simulink model "CLLC_simu"  (R2025b)
settings: Solver=ode23tb  StartTime=0.0  StopTime=simlength  MaxStep=tc  RelTol=1e-3
values from neighbouring files (symbols this model uses):
  alpha1 = 0    [init.m]    (also in state_space_equations.m = linspace(pi/2,pi,3))
  alpha2 = 0    [init.m]    (also in state_space_equations.m = linspace(pi/2,pi,3))
  fr = 1/(2*pi*sqrt(Lr1*Cr1))    [init.m]
  phase_shift = pi/6    (= 0.523598775598)    [init.m]
  R1 = 0.026    [Optimal_Design_CLLLC.m]    (also in init.m = 0.1; state_space_equations.m = 0.1)
  R2 = 0.026    [Optimal_Design_CLLLC.m]    (also in init.m = 0.1; state_space_equations.m = 0.1)
  Td = 0.015 * Ts    (= 1.66666666667e-07)    [init.m]
libraries: fl_lib x60, nesl_utility x35, ee_lib x2, eeGeneralControl x1, single_phase_transformer x1
(part 1 of 2)
settings Model: SimulationMode=accelerator  Creator=i0013805  LastModifiedBy=torai

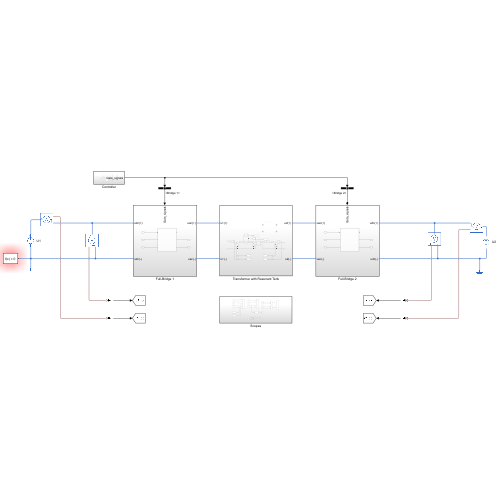
[thumbnail: Simulink's stored preview of the top-level diagram]
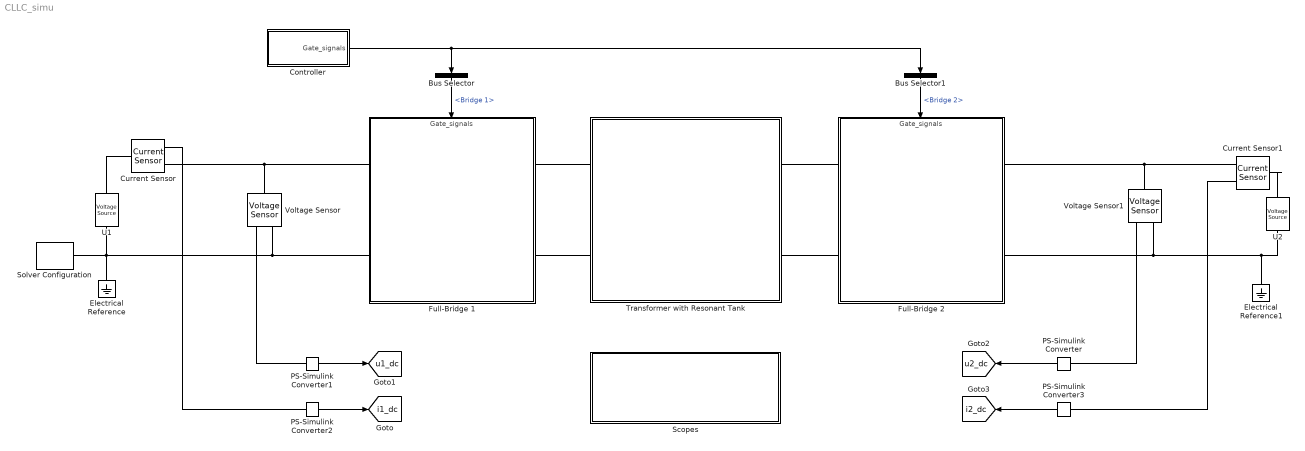
== system CLLC_simu ==
  Bus Selector : BusSelector  OutputSignals=Bridge 1
  Bus Selector1 : BusSelector  OutputSignals=Bridge 2
  Controller : Subsystem
  Current Sensor : fl_lib/Electrical/Electrical Sensors/Current Sensor
  Current Sensor1 : fl_lib/Electrical/Electrical Sensors/Current Sensor
  Electrical Reference : fl_lib/Electrical/Electrical Elements/Electrical Reference
  Electrical Reference1 : fl_lib/Electrical/Electrical Elements/Electrical Reference
  Full-Bridge 1 : Subsystem
      settings: PortSchema="{\"entries\":[{\"content\":{\"sides\":[{\"content\":{\"connectorIds\":[\"LConn1\",\"LConn2\"]},\"type\":\"ConnectorPlacement.EquallySpacedRectSide\",\"uuid\":\"3353105e-e30e-4d15-8630-1aa6d339e0ff\"},{\"content\":{\"connectorIds\":[\"RConn1\",\"RConn2\"],\"side\":\"RIGHT\"},\"type\":\"ConnectorPlacement.EquallySpacedRectSide\",\"uuid\":\"296f84bb-4176-46a6-993d-d3f03b5e0e3a\"},{\"content\":{\"connectorIds\":[\"In1\"],\"side\":\"TOP\"},\"type\":\"ConnectorPlacement.EquallySpacedRectSide\",\"uuid\":\"5e45aedc-9cf5-4fc9-baa6-17227fc5f4f5\"}]},\"type\":\"ConnectorPlacement.EquallySpacedConnector\",\"uuid\":\"c9e49bb0-57c4-4cc0-be60-b6700ac8c03a\"}],\"packageUris\":[\"http://schema.mathworks.com/mf0/Connector/R2020b\"],\"version\":\"1.0\"}"
  Full-Bridge 2 : Subsystem
      settings: PortSchema="{\"entries\":[{\"content\":{\"sides\":[{\"content\":{\"connectorIds\":[\"LConn1\",\"LConn2\"]},\"type\":\"ConnectorPlacement.EquallySpacedRectSide\",\"uuid\":\"3353105e-e30e-4d15-8630-1aa6d339e0ff\"},{\"content\":{\"connectorIds\":[\"RConn1\",\"RConn2\"],\"side\":\"RIGHT\"},\"type\":\"ConnectorPlacement.EquallySpacedRectSide\",\"uuid\":\"296f84bb-4176-46a6-993d-d3f03b5e0e3a\"},{\"content\":{\"connectorIds\":[\"In1\"],\"side\":\"TOP\"},\"type\":\"ConnectorPlacement.EquallySpacedRectSide\",\"uuid\":\"5e45aedc-9cf5-4fc9-baa6-17227fc5f4f5\"}]},\"type\":\"ConnectorPlacement.EquallySpacedConnector\",\"uuid\":\"c9e49bb0-57c4-4cc0-be60-b6700ac8c03a\"}],\"packageUris\":[\"http://schema.mathworks.com/mf0/Connector/R2020b\"],\"version\":\"1.0\"}"
  PS-Simulink Converter{,1..3} (4 alike) : nesl_utility/PS-Simulink Converter  PhysicalDomain=network_engine_domain  SubClassName=ps_output  LeftPortType=input  RightPortType=output  PseudoPeriodic=off  Frequencies=[]  VectorFormat=inherit  Unit=inherit  AffineConversion=off
  Scopes : Subsystem
  Solver Configuration : nesl_utility/Solver Configuration  PhysicalDomain=network_engine_domain  SubClassName=solver  LeftPortType=input  RightPortType=generic  Tones=[]  Harmonics=[]  SimulateNoise=off  Profile=off  UseLocalSampling=off  EnableSwitchedLinearOptims=on  FrequencyDomain=off  UseCCode=off  RelTol=0.001  AbsTol=0.001  MinStep=1e-09  ToWorkspace=off  RevertToSquareIcSolve=off  NumHomotopyIterations=100  PhasorMode=off  PhasorModeNumHarmonics=1  ConsistencySolver=NEWTON_XTOL_AFTER_FTOL  IndexReductionMethod=DerivativeReplacement  DoDC=off  ResidualTolerance=1e-09  ConsistencyTolSource=GLOBAL  ConsistencyAbsTol=0.001  ConsistencyRelTol=0.001  ConsistencyTolFactor=0.001  UseLocalSolver=on  LocalSolverChoice=NE_BACKWARD_EULER_ADVANCER  ResolveIndetEquations=on  FunctionEvalNumThread=1  LocalSolverSampleTime=tc  DoFixedCost=on  MaxNonlinIter=5  MaxModeIter=2  ComputeImpulses=off  ImpulseIterations=2  LinearAlgebra=auto  LinearAlgebraNumThread=0  EquationFormulation=NE_TIME_EF  DelaysMemoryBudget=1024  AutomaticFiltering=on  FilteringTimeConstant=0.001  PartitionStorageMethod=AS_NEEDED  PartitionMemoryBudget=1024  PartitionMethod=ROBUST  MultibodyUseLocalSolver=off  MultibodyLocalSolverChoice=ODE1  MultibodyLocalSolverSampleTime=0.001
  Transformer with Resonant Tank : Subsystem
  U1 : ee_lib/Sources/Voltage Source  dc_voltage=800 V  ac_voltage=0 V  ac_shift=0 rad  ac_frequency=60 Hz  noise_mode=ee.enum.sources.noise.Disabled  PSD=0 V^2/Hz  sample_time=1e-3 s  repeatability=ee.enum.sources.repeatability.NotRepeatable  user_seed=0  auto_seed=3499211588  i_specify=off  i_priority=None  i=0 A  i_nominal_specify=off  i_nominal_value=1  i_nominal_unit=A  v_specify=off  v_priority=None  v=0 V  v_nominal_specify=off  v_nominal_value=1  v_nominal_unit=V
  U2 : ee_lib/Sources/Voltage Source  dc_voltage=800 V  ac_voltage=0 V  ac_shift=0 rad  ac_frequency=60 Hz  noise_mode=ee.enum.sources.noise.Disabled  PSD=0 V^2/Hz  sample_time=1e-3 s  repeatability=ee.enum.sources.repeatability.NotRepeatable  user_seed=0  auto_seed=3890346746  i_specify=off  i_priority=None  i=0 A  i_nominal_specify=off  i_nominal_value=1  i_nominal_unit=A  v_specify=off  v_priority=None  v=0 V  v_nominal_specify=off  v_nominal_value=1  v_nominal_unit=V
  Voltage Sensor : fl_lib/Electrical/Electrical Sensors/Voltage Sensor
  Voltage Sensor1 : fl_lib/Electrical/Electrical Sensors/Voltage Sensor
  tag scope: i1_dc=global, i2_dc=global, u1_dc=global, u2_dc=global
  wires:
  Bus Selector/1 -> Full-Bridge 1/1(Gate_signals)  "<Bridge 1>"
  Controller/1(Gate_signals) -> Bus Selector1/1, Bus Selector/1
  Bus Selector1/1 -> Full-Bridge 2/1(Gate_signals)  "<Bridge 2>"
  PS-Simulink Converter2/1 -> [i1_dc]
  PS-Simulink Converter1/1 -> [u1_dc]
  PS-Simulink Converter/1 -> [u2_dc]
  PS-Simulink Converter3/1 -> [i2_dc]
  connections:
  U2/RConn1 -- Electrical Reference1/LConn1 -- Full-Bridge 2/LConn2 -- Voltage Sensor1/RConn2
  Voltage Sensor/LConn1 -- Current Sensor/RConn2 -- Full-Bridge 1/LConn1
  Full-Bridge 1/RConn1 -- Transformer with Resonant Tank/LConn1
  Full-Bridge 1/RConn2 -- Transformer with Resonant Tank/LConn2
  U1/RConn1 -- Electrical Reference/LConn1 -- Full-Bridge 1/LConn2 -- Voltage Sensor/RConn2 -- Solver Configuration/RConn1
  Voltage Sensor/RConn1 -- PS-Simulink Converter1/LConn1
  Voltage Sensor1/RConn1 -- PS-Simulink Converter/LConn1
  Current Sensor/LConn1 -- U1/LConn1
  PS-Simulink Converter2/LConn1 -- Current Sensor/RConn1
  PS-Simulink Converter3/LConn1 -- Current Sensor1/RConn1
  Full-Bridge 2/RConn1 -- Transformer with Resonant Tank/RConn1
  Transformer with Resonant Tank/RConn2 -- Full-Bridge 2/RConn2
  Current Sensor1/LConn1 -- U2/LConn1
  Full-Bridge 2/LConn1 -- Current Sensor1/RConn2 -- Voltage Sensor1/LConn1

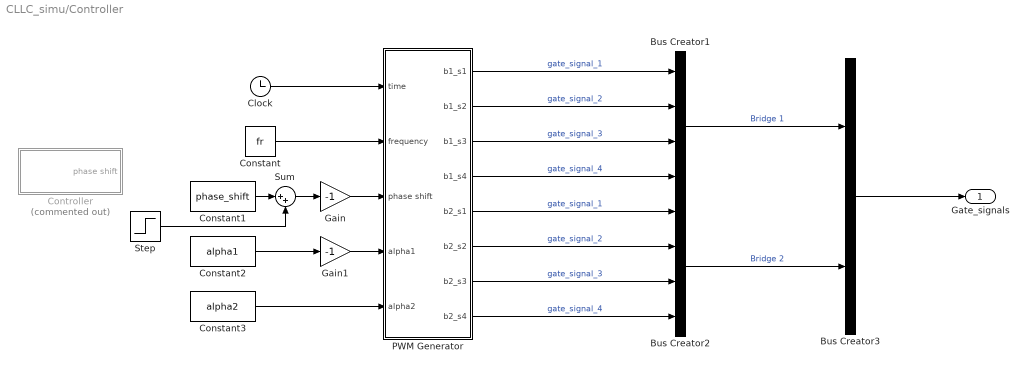
== system CLLC_simu/Controller ==
  Bus Creator1 : BusCreator  Inputs=4
  Bus Creator2 : BusCreator  Inputs=4
  Bus Creator3 : BusCreator  Inputs=2
  Clock : Clock
  Constant : Constant  Value=fr  VectorParams1D=off
  Constant1 : Constant  Value=phase_shift
  Constant2 : Constant  Value=alpha1
  Constant3 : Constant  Value=alpha2
  Controller : Subsystem  Commented=on
  Gain : Gain  Gain=-1
  Gain1 : Gain  Gain=-1
  PWM Generator : Subsystem
  Step : Step  Time=0.3  After=2*pi*0.04  SampleTime=0
  Sum : Sum  Inputs=|++
  Gate_signals : Outport
  wires:
  Bus Creator3/1 -> Gate_signals/1
  Bus Creator1/1 -> Bus Creator3/1  "Bridge 1"
  Bus Creator2/1 -> Bus Creator3/2  "Bridge 2"
  PWM Generator/1(b1_s1) -> Bus Creator1/1  "gate_signal_1"
  PWM Generator/4(b1_s4) -> Bus Creator1/4  "gate_signal_4"
  PWM Generator/2(b1_s2) -> Bus Creator1/2  "gate_signal_2"
  PWM Generator/3(b1_s3) -> Bus Creator1/3  "gate_signal_3"
  PWM Generator/5(b2_s1) -> Bus Creator2/1  "gate_signal_1"
  PWM Generator/6(b2_s2) -> Bus Creator2/2  "gate_signal_2"
  PWM Generator/7(b2_s3) -> Bus Creator2/3  "gate_signal_3"
  PWM Generator/8(b2_s4) -> Bus Creator2/4  "gate_signal_4"
  Clock/1 -> PWM Generator/1(time)
  Constant/1 -> PWM Generator/2(frequency)
  Constant2/1 -> Gain1/1
  Constant3/1 -> PWM Generator/5(alpha2)
  Gain/1 -> PWM Generator/3(phase shift)
  Gain1/1 -> PWM Generator/4(alpha1)
  Constant1/1 -> Sum/1
  Sum/1 -> Gain/1
  Step/1 -> Sum/2

== system CLLC_simu/Full-Bridge 1 ==
  Gate_signals : Inport
  Full-Bridge Ideal Switches : Subsystem
  udc(+) : PMIOPort  Side=Left
  udc(-) : PMIOPort  Port=2  Side=Left
  uac(+) : PMIOPort  Port=3  Side=Right
  uac(-) : PMIOPort  Port=4  Side=Right
  wires:
  Gate_signals/1 -> Full-Bridge Ideal Switches/1(Gate_signals)
  connections:
  udc(-)/RConn1 -- Full-Bridge Ideal Switches/LConn2
  Full-Bridge Ideal Switches/RConn1 -- uac(+)/RConn1
  Full-Bridge Ideal Switches/RConn2 -- uac(-)/RConn1
  udc(+)/RConn1 -- Full-Bridge Ideal Switches/LConn1

== system CLLC_simu/Full-Bridge 2 ==
  Gate_signals : Inport
  Full-Bridge Ideal Switches : Subsystem
  udc(+) : PMIOPort  Side=Left
  udc(-) : PMIOPort  Port=2  Side=Left
  uac(+) : PMIOPort  Port=3  Side=Right
  uac(-) : PMIOPort  Port=4  Side=Right
  wires:
  Gate_signals/1 -> Full-Bridge Ideal Switches/1(Gate_signals)
  connections:
  udc(-)/RConn1 -- Full-Bridge Ideal Switches/LConn2
  Full-Bridge Ideal Switches/RConn1 -- uac(+)/RConn1
  Full-Bridge Ideal Switches/RConn2 -- uac(-)/RConn1
  udc(+)/RConn1 -- Full-Bridge Ideal Switches/LConn1

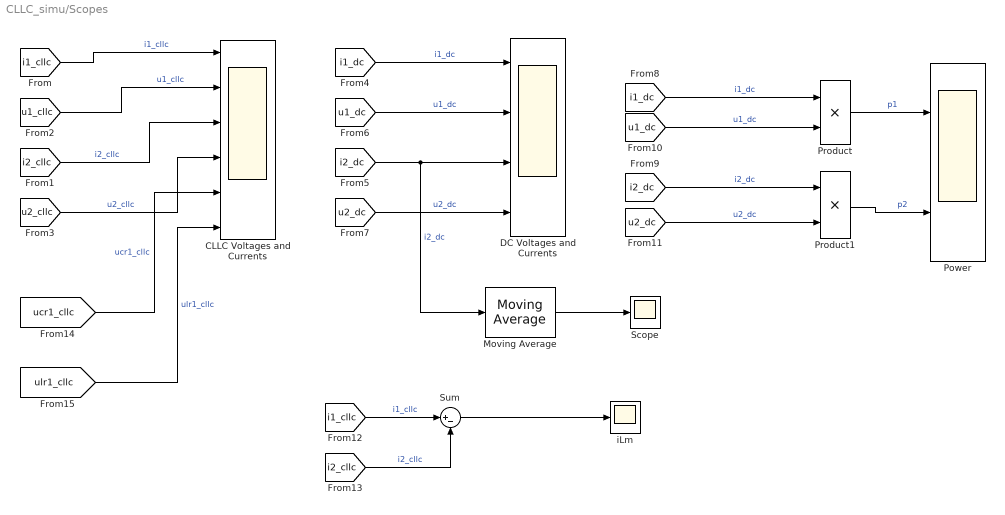
== system CLLC_simu/Scopes ==
  CLLC Voltages and Currents : Scope  NumInputPorts=6
      settings: ActiveDisplayYMinimum=-1023.9248688451665  ActiveDisplayYMaximum=1024.1887494959194
  DC Voltages and Currents : Scope  NumInputPorts=4
      settings: ActiveDisplayString=4  ActiveDisplayYMinimum=9  ActiveDisplayYMaximum=29
  Moving Average : eeGeneralControl/Moving Average  VariantControl=Variant1  LabelModeActiveChoice=Discrete  f=100e3  x0=0  BufferSize=8192  Ts=-1
      settings: LibrarySourceBlock=ee_sl_lib/General Control/Moving Average
  Power : Scope  NumInputPorts=2
      settings: ActiveDisplayYMinimum=-2.5651019732390419E+6  ActiveDisplayYMaximum=1.2445984514162283E+7  DataLoggingVariableName=ScopeData2
  Product : Product
  Product1 : Product
  Scope : Scope
      settings: ActiveDisplayYMinimum=-3.0858146971641012  ActiveDisplayYMaximum=-1.209999064201392  DataLoggingVariableName=ScopeData4
  Sum : Sum  Inputs=|+-
  iLm : Scope
      settings: ActiveDisplayYMinimum=-41.350666404493246  ActiveDisplayYMaximum=41.348326835244379  DataLoggingVariableName=ScopeData3
  wires:
  [i1_cllc] -> CLLC Voltages and Currents/1  "i1_cllc"
  [u1_cllc] -> CLLC Voltages and Currents/2  "u1_cllc"
  [i2_cllc] -> CLLC Voltages and Currents/3  "i2_cllc"
  [u2_cllc] -> CLLC Voltages and Currents/4  "u2_cllc"
  [i1_dc] -> DC Voltages and Currents/1  "i1_dc"
  [u1_dc] -> DC Voltages and Currents/2  "u1_dc"
  [i2_dc] -> Moving Average/1, DC Voltages and Currents/3  "i2_dc"
  [u2_dc] -> DC Voltages and Currents/4  "u2_dc"
  [i1_dc] -> Product/1  "i1_dc"
  [i2_dc] -> Product1/1  "i2_dc"
  [u1_dc] -> Product/2  "u1_dc"
  Product/1 -> Power/1  "p1"
  Product1/1 -> Power/2  "p2"
  [u2_dc] -> Product1/2  "u2_dc"
  [i1_cllc] -> Sum/1  "i1_cllc"
  [i2_cllc] -> Sum/2  "i2_cllc"
  Sum/1 -> iLm/1
  Moving Average/1 -> Scope/1
  [ucr1_cllc] -> CLLC Voltages and Currents/5  "ucr1_cllc"
  [ulr1_cllc] -> CLLC Voltages and Currents/6  "ulr1_cllc"

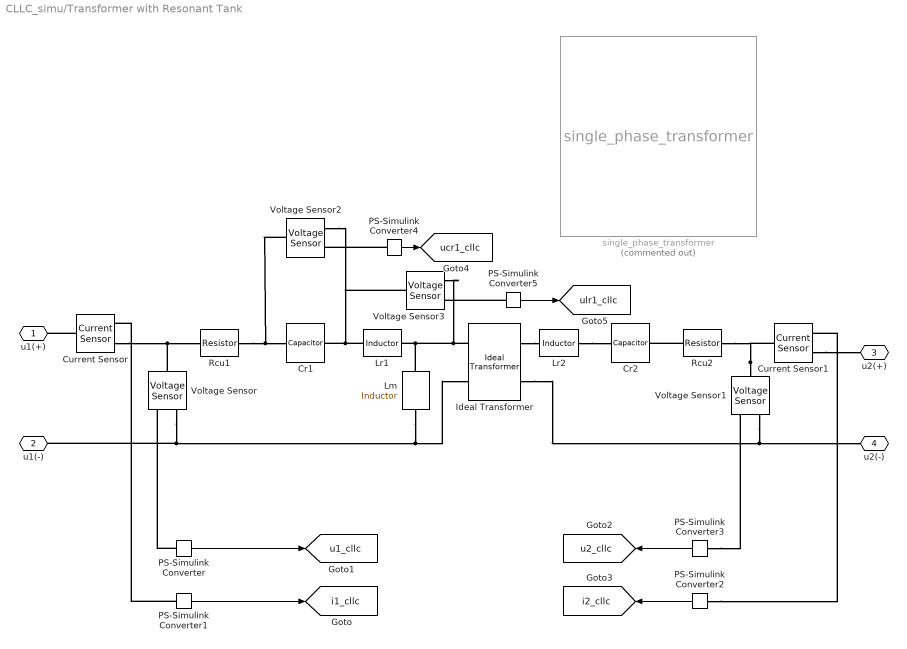
== system CLLC_simu/Transformer with Resonant Tank ==
  Cr1 : fl_lib/Electrical/Electrical Elements/Capacitor  c=Cr1 F  r=1e-6 Ohm  g=0 1/Ohm  i_specify=off  i_priority=None  i=0 A  i_nominal_specify=off  i_nominal_value=1  i_nominal_unit=A  v_specify=off  v_priority=None  v=0 V  v_nominal_specify=off  v_nominal_value=1  v_nominal_unit=V  vc_specify=off  vc_priority=High  vc=0 V  vc_nominal_specify=off  vc_nominal_value=1  vc_nominal_unit=V
  Cr2 : fl_lib/Electrical/Electrical Elements/Capacitor  c=Cr2 F  r=1e-6 Ohm  g=0 1/Ohm  i_specify=off  i_priority=None  i=0 A  i_nominal_specify=off  i_nominal_value=1  i_nominal_unit=A  v_specify=off  v_priority=None  v=0 V  v_nominal_specify=off  v_nominal_value=1  v_nominal_unit=V  vc_specify=off  vc_priority=High  vc=0 V  vc_nominal_specify=off  vc_nominal_value=1  vc_nominal_unit=V
  Current Sensor : fl_lib/Electrical/Electrical Sensors/Current Sensor
  Current Sensor1 : fl_lib/Electrical/Electrical Sensors/Current Sensor
  Ideal Transformer : fl_lib/Electrical/Electrical Elements/Ideal Transformer  n=1  i1_specify=off  i1_priority=None  i1=0 A  i1_nominal_specify=off  i1_nominal_value=1  i1_nominal_unit=A  v1_specify=off  v1_priority=None  v1=0 V  v1_nominal_specify=off  v1_nominal_value=1  v1_nominal_unit=V  i2_specify=off  i2_priority=None  i2=0 A  i2_nominal_specify=off  i2_nominal_value=1  i2_nominal_unit=A  v2_specify=off  v2_priority=None  v2=0 V  v2_nominal_specify=off  v2_nominal_value=1  v2_nominal_unit=V
  Lm : fl_lib/Electrical/Electrical Elements/Inductor  l=Lm H  r=0 Ohm  g=1e-9 1/Ohm  i_specify=off  i_priority=None  i=0 A  i_nominal_specify=off  i_nominal_value=1  i_nominal_unit=A  v_specify=off  v_priority=None  v=0 V  v_nominal_specify=off  v_nominal_value=1  v_nominal_unit=V  i_L_specify=off  i_L_priority=High  i_L=0 A  i_L_nominal_specify=off  i_L_nominal_value=1  i_L_nominal_unit=A
  Lr1 : fl_lib/Electrical/Electrical Elements/Inductor  l=Lr1 H  r=0 Ohm  g=1e-9 1/Ohm  i_specify=off  i_priority=None  i=0 A  i_nominal_specify=off  i_nominal_value=1  i_nominal_unit=A  v_specify=off  v_priority=None  v=0 V  v_nominal_specify=off  v_nominal_value=1  v_nominal_unit=V  i_L_specify=off  i_L_priority=High  i_L=0 A  i_L_nominal_specify=off  i_L_nominal_value=1  i_L_nominal_unit=A
  Lr2 : fl_lib/Electrical/Electrical Elements/Inductor  l=Lr2 H  r=0 Ohm  g=1e-9 1/Ohm  i_specify=off  i_priority=None  i=0 A  i_nominal_specify=off  i_nominal_value=1  i_nominal_unit=A  v_specify=off  v_priority=None  v=0 V  v_nominal_specify=off  v_nominal_value=1  v_nominal_unit=V  i_L_specify=off  i_L_priority=High  i_L=0 A  i_L_nominal_specify=off  i_L_nominal_value=1  i_L_nominal_unit=A
  PS-Simulink Converter{,1..5} (6 alike) : nesl_utility/PS-Simulink Converter  PhysicalDomain=network_engine_domain  SubClassName=ps_output  LeftPortType=input  RightPortType=output  PseudoPeriodic=off  Frequencies=[]  VectorFormat=inherit  Unit=inherit  AffineConversion=off
  Rcu1 : fl_lib/Electrical/Electrical Elements/Resistor  R=R1 Ohm  i_specify=off  i_priority=None  i=0 A  i_nominal_specify=off  i_nominal_value=1  i_nominal_unit=A  v_specify=off  v_priority=None  v=0 V  v_nominal_specify=off  v_nominal_value=1  v_nominal_unit=V
  Rcu2 : fl_lib/Electrical/Electrical Elements/Resistor  R=R2 Ohm  i_specify=off  i_priority=None  i=0 A  i_nominal_specify=off  i_nominal_value=1  i_nominal_unit=A  v_specify=off  v_priority=None  v=0 V  v_nominal_specify=off  v_nominal_value=1  v_nominal_unit=V
  Voltage Sensor{,1..3} (4 alike) : fl_lib/Electrical/Electrical Sensors/Voltage Sensor
  single_phase_transformer : single_phase_transformer/single_phase_transformer  Commented=on  lm_trafo=L_m  m1=N1  m2=N2  rd1_trafo=R1  rd2_trafo=R2  ld1_trafo=Lr1  ld2_trafo=Lr2  rfe_trafo=Rfe  length_core=0.1  mu0=1.256637e-6  mur=mur
  u1(+) : PMIOPort  Side=Left
  u1(-) : PMIOPort  Port=2  Side=Left
  u2(+) : PMIOPort  Port=3  Side=Right
  u2(-) : PMIOPort  Port=4  Side=Right
  tag scope: i1_cllc=global, i2_cllc=global, u1_cllc=global, u2_cllc=global, ucr1_cllc=global, ulr1_cllc=global
  wires:
  PS-Simulink Converter1/1 -> [i1_cllc]
  PS-Simulink Converter/1 -> [u1_cllc]
  PS-Simulink Converter3/1 -> [u2_cllc]
  PS-Simulink Converter2/1 -> [i2_cllc]
  PS-Simulink Converter4/1 -> [ucr1_cllc]
  PS-Simulink Converter5/1 -> [ulr1_cllc]
  connections:
  Lr2/RConn1 -- Cr2/RConn1
  Lr1/LConn1 -- Voltage Sensor3/LConn1 -- Voltage Sensor2/RConn2 -- Cr1/RConn1
  Voltage Sensor1/RConn2 -- Ideal Transformer/RConn2 -- u2(-)/RConn1
  Voltage Sensor/LConn1 -- Current Sensor/RConn2 -- Rcu1/LConn1
  Voltage Sensor/RConn2 -- Lm/RConn1 -- Ideal Transformer/LConn2 -- u1(-)/RConn1
  Rcu2/RConn1 -- Cr2/LConn1
  PS-Simulink Converter/LConn1 -- Voltage Sensor/RConn1
  Current Sensor/LConn1 -- u1(+)/RConn1
  PS-Simulink Converter1/LConn1 -- Current Sensor/RConn1
  Current Sensor1/RConn2 -- u2(+)/RConn1
  PS-Simulink Converter3/LConn1 -- Voltage Sensor1/RConn1
  PS-Simulink Converter2/LConn1 -- Current Sensor1/RConn1
  Ideal Transformer/LConn1 -- Voltage Sensor3/RConn2 -- Lm/LConn1 -- Lr1/RConn1
  Ideal Transformer/RConn1 -- Lr2/LConn1
  PS-Simulink Converter4/LConn1 -- Voltage Sensor2/RConn1
  PS-Simulink Converter5/LConn1 -- Voltage Sensor3/RConn1
  Rcu1/RConn1 -- Voltage Sensor2/LConn1 -- Cr1/LConn1
  Voltage Sensor1/LConn1 -- Current Sensor1/LConn1 -- Rcu2/LConn1

== system CLLC_simu/Controller/Controller ==
  Constant : Constant
  Gain : Gain  Gain=1/(200e3/800)
  Gain1 : Gain  Gain=-1
  Quantizer : Quantizer  QuantizationInterval=0.00048828
  Subsystem : Subsystem
  Sum : Sum  Inputs=|+-
  Unit Delay2 : UnitDelay  SampleTime=-1  HasFrameUpgradeWarning=on
  Zero-Order Hold2 : ZeroOrderHold  SampleTime=-1
  phase shift : Outport
  wires:
  Constant/1 -> Sum/1
  [i2_dc] -> Gain/1
  Gain/1 -> Quantizer/1
  Quantizer/1 -> Zero-Order Hold2/1
  Zero-Order Hold2/1 -> Sum/2
  Gain1/1 -> Unit Delay2/1
  Sum/1 -> Subsystem/1(In1)
  Subsystem/1(Out1) -> Gain1/1
  Unit Delay2/1 -> phase shift/1

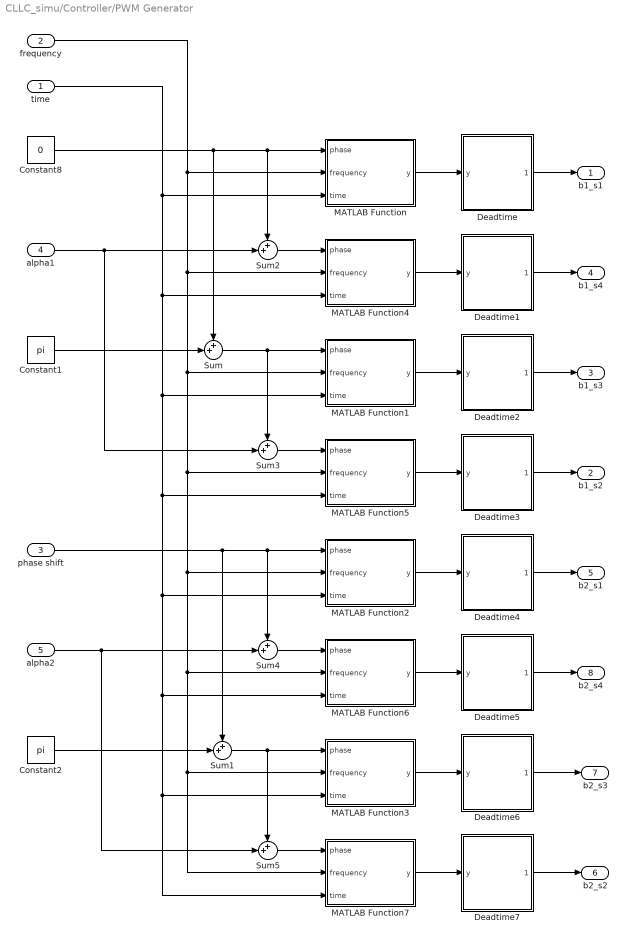
== system CLLC_simu/Controller/PWM Generator ==
  time : Inport
  frequency : Inport  Port=2
  phase shift : Inport  Port=3
  alpha1 : Inport  Port=4
  alpha2 : Inport  Port=5
  Constant1 : Constant  Value=pi
  Constant2 : Constant  Value=pi
  Constant8 : Constant  Value=0
  Deadtime : Subsystem
  Deadtime1 : Subsystem
  Deadtime2 : Subsystem
  Deadtime3 : Subsystem
  Deadtime4 : Subsystem
  Deadtime5 : Subsystem
  Deadtime6 : Subsystem
  Deadtime7 : Subsystem
  MATLAB Function : MATLAB Function  TreatAsAtomicUnit=on
  MATLAB Function1 : MATLAB Function  TreatAsAtomicUnit=on
  MATLAB Function2 : MATLAB Function  TreatAsAtomicUnit=on
  MATLAB Function3 : MATLAB Function  TreatAsAtomicUnit=on
  MATLAB Function4 : MATLAB Function  TreatAsAtomicUnit=on
  MATLAB Function5 : MATLAB Function  TreatAsAtomicUnit=on
  MATLAB Function6 : MATLAB Function  TreatAsAtomicUnit=on
  MATLAB Function7 : MATLAB Function  TreatAsAtomicUnit=on
  Sum{,1..5} (6 alike) : Sum  Inputs=++|
  b1_s1 : Outport
  b1_s2 : Outport  Port=2
  b1_s3 : Outport  Port=3
  b1_s4 : Outport  Port=4
  b2_s1 : Outport  Port=5
  b2_s2 : Outport  Port=6
  b2_s3 : Outport  Port=7
  b2_s4 : Outport  Port=8
  wires:
  Constant8/1 -> Sum/1, Sum2/1, MATLAB Function/1(phase)
  frequency/1 -> MATLAB Function5/2(frequency), MATLAB Function7/2(frequency), MATLAB Function3/2(frequency), MATLAB Function6/2(frequency), MATLAB Function2/2(frequency), MATLAB Function1/2(frequency), MATLAB Function4/2(frequency), MATLAB Function/2(frequency)
  time/1 -> MATLAB Function5/3(time), MATLAB Function3/3(time), MATLAB Function7/3(time), MATLAB Function6/3(time), MATLAB Function2/3(time), MATLAB Function1/3(time), MATLAB Function4/3(time), MATLAB Function/3(time)
  Sum/1 -> MATLAB Function1/1(phase), Sum3/1
  phase shift/1 -> Sum1/1, Sum4/1, MATLAB Function2/1(phase)
  Sum1/1 -> Sum5/1, MATLAB Function3/1(phase)
  MATLAB Function/1(y) -> Deadtime/1(y)
  Deadtime/1(1) -> b1_s1/1
  MATLAB Function1/1(y) -> Deadtime2/1(y)
  MATLAB Function2/1(y) -> Deadtime4/1(y)
  Deadtime5/1(1) -> b2_s4/1
  MATLAB Function3/1(y) -> Deadtime6/1(y)
  Deadtime6/1(1) -> b2_s3/1
  Deadtime7/1(1) -> b2_s2/1
  Constant1/1 -> Sum/2
  Constant2/1 -> Sum1/2
  Deadtime3/1(1) -> b1_s2/1
  alpha1/1 -> Sum3/2, Sum2/2
  Sum2/1 -> MATLAB Function4/1(phase)
  MATLAB Function4/1(y) -> Deadtime1/1(y)
  Deadtime1/1(1) -> b1_s4/1
  Sum3/1 -> MATLAB Function5/1(phase)
  MATLAB Function5/1(y) -> Deadtime3/1(y)
  Deadtime2/1(1) -> b1_s3/1
  Sum4/1 -> MATLAB Function6/1(phase)
  alpha2/1 -> Sum5/2, Sum4/2
  Deadtime4/1(1) -> b2_s1/1
  MATLAB Function6/1(y) -> Deadtime5/1(y)
  MATLAB Function7/1(y) -> Deadtime7/1(y)
  Sum5/1 -> MATLAB Function7/1(phase)

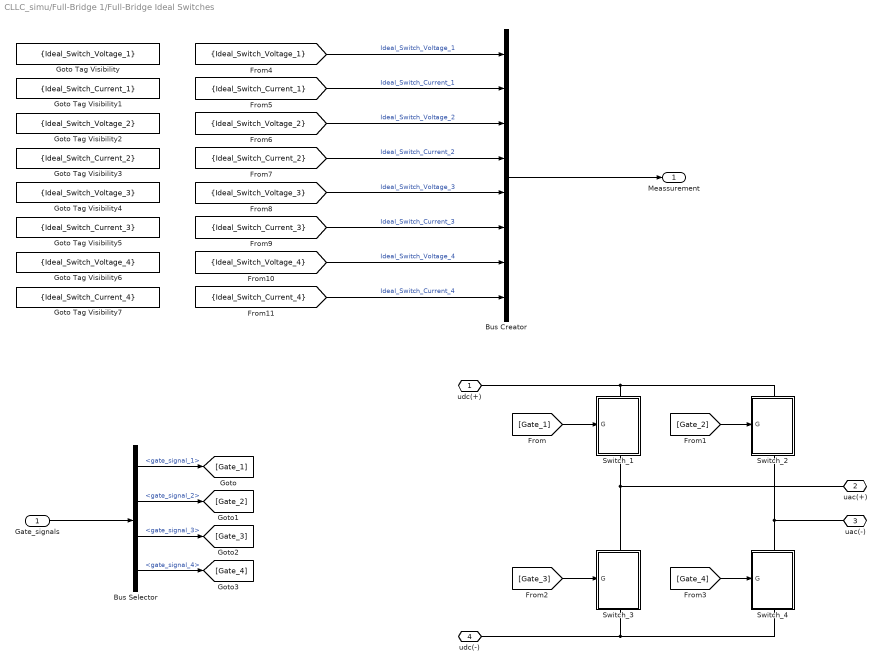
== system CLLC_simu/Full-Bridge 1/Full-Bridge Ideal Switches ==
  Gate_signals : Inport
  Bus Creator : BusCreator  Inputs=8
  Bus Selector : BusSelector  OutputSignals=gate_signal_1,gate_signal_2,gate_signal_3,gate_signal_4
  Goto Tag Visibility : GotoTagVisibility  GotoTag=Ideal_Switch_Voltage_1
  Goto Tag Visibility1 : GotoTagVisibility  GotoTag=Ideal_Switch_Current_1
  Goto Tag Visibility2 : GotoTagVisibility  GotoTag=Ideal_Switch_Voltage_2
  Goto Tag Visibility3 : GotoTagVisibility  GotoTag=Ideal_Switch_Current_2
  Goto Tag Visibility4 : GotoTagVisibility  GotoTag=Ideal_Switch_Voltage_3
  Goto Tag Visibility5 : GotoTagVisibility  GotoTag=Ideal_Switch_Current_3
  Goto Tag Visibility6 : GotoTagVisibility  GotoTag=Ideal_Switch_Voltage_4
  Goto Tag Visibility7 : GotoTagVisibility  GotoTag=Ideal_Switch_Current_4
  Switch_1 : Subsystem
      settings: PortSchema="{\"entries\":[{\"content\":{\"sides\":[{\"content\":{\"connectorIds\":[\"In1\"]},\"type\":\"ConnectorPlacement.EquallySpacedRectSide\",\"uuid\":\"812df248-72cf-4017-9d54-aef7207fce7f\"},{\"content\":{\"side\":\"RIGHT\"},\"type\":\"ConnectorPlacement.EquallySpacedRectSide\",\"uuid\":\"a66e31eb-6559-4312-afa0-26cb116d02bf\"},{\"content\":{\"connectorIds\":[\"LConn1\"],\"side\":\"TOP\"},\"type\":\"ConnectorPlacement.EquallySpacedRectSide\",\"uuid\":\"1df6feb4-8a8d-441a-a0dc-721a2bb21abb\"},{\"content\":{\"connectorIds\":[\"RConn1\"],\"side\":\"BOTTOM\"},\"type\":\"ConnectorPlacement.EquallySpacedRectSide\",\"uuid\":\"258c1e92-2fe7-4acf-9dd0-9c6d3fd42034\"}]},\"type\":\"ConnectorPlacement.EquallySpacedConnector\",\"uuid\":\"c9b0d122-031a-4b9b-b90c-c03d042c7b1a\"}],\"packageUris\":[\"http://schema.mathworks.com/mf0/Connector/R2020b\"],\"version\":\"1.0\"}"
  Switch_2 : Subsystem
      settings: PortSchema="{\"entries\":[{\"content\":{\"sides\":[{\"content\":{\"connectorIds\":[\"In1\"]},\"type\":\"ConnectorPlacement.EquallySpacedRectSide\",\"uuid\":\"812df248-72cf-4017-9d54-aef7207fce7f\"},{\"content\":{\"side\":\"RIGHT\"},\"type\":\"ConnectorPlacement.EquallySpacedRectSide\",\"uuid\":\"a66e31eb-6559-4312-afa0-26cb116d02bf\"},{\"content\":{\"connectorIds\":[\"LConn1\"],\"side\":\"TOP\"},\"type\":\"ConnectorPlacement.EquallySpacedRectSide\",\"uuid\":\"1df6feb4-8a8d-441a-a0dc-721a2bb21abb\"},{\"content\":{\"connectorIds\":[\"RConn1\"],\"side\":\"BOTTOM\"},\"type\":\"ConnectorPlacement.EquallySpacedRectSide\",\"uuid\":\"258c1e92-2fe7-4acf-9dd0-9c6d3fd42034\"}]},\"type\":\"ConnectorPlacement.EquallySpacedConnector\",\"uuid\":\"c9b0d122-031a-4b9b-b90c-c03d042c7b1a\"}],\"packageUris\":[\"http://schema.mathworks.com/mf0/Connector/R2020b\"],\"version\":\"1.0\"}"
  Switch_3 : Subsystem
      settings: PortSchema="{\"entries\":[{\"content\":{\"sides\":[{\"content\":{\"connectorIds\":[\"In1\"]},\"type\":\"ConnectorPlacement.EquallySpacedRectSide\",\"uuid\":\"812df248-72cf-4017-9d54-aef7207fce7f\"},{\"content\":{\"side\":\"RIGHT\"},\"type\":\"ConnectorPlacement.EquallySpacedRectSide\",\"uuid\":\"a66e31eb-6559-4312-afa0-26cb116d02bf\"},{\"content\":{\"connectorIds\":[\"LConn1\"],\"side\":\"TOP\"},\"type\":\"ConnectorPlacement.EquallySpacedRectSide\",\"uuid\":\"1df6feb4-8a8d-441a-a0dc-721a2bb21abb\"},{\"content\":{\"connectorIds\":[\"RConn1\"],\"side\":\"BOTTOM\"},\"type\":\"ConnectorPlacement.EquallySpacedRectSide\",\"uuid\":\"258c1e92-2fe7-4acf-9dd0-9c6d3fd42034\"}]},\"type\":\"ConnectorPlacement.EquallySpacedConnector\",\"uuid\":\"c9b0d122-031a-4b9b-b90c-c03d042c7b1a\"}],\"packageUris\":[\"http://schema.mathworks.com/mf0/Connector/R2020b\"],\"version\":\"1.0\"}"
  Switch_4 : Subsystem
      settings: PortSchema="{\"entries\":[{\"content\":{\"sides\":[{\"content\":{\"connectorIds\":[\"In1\"]},\"type\":\"ConnectorPlacement.EquallySpacedRectSide\",\"uuid\":\"812df248-72cf-4017-9d54-aef7207fce7f\"},{\"content\":{\"side\":\"RIGHT\"},\"type\":\"ConnectorPlacement.EquallySpacedRectSide\",\"uuid\":\"a66e31eb-6559-4312-afa0-26cb116d02bf\"},{\"content\":{\"connectorIds\":[\"LConn1\"],\"side\":\"TOP\"},\"type\":\"ConnectorPlacement.EquallySpacedRectSide\",\"uuid\":\"1df6feb4-8a8d-441a-a0dc-721a2bb21abb\"},{\"content\":{\"connectorIds\":[\"RConn1\"],\"side\":\"BOTTOM\"},\"type\":\"ConnectorPlacement.EquallySpacedRectSide\",\"uuid\":\"258c1e92-2fe7-4acf-9dd0-9c6d3fd42034\"}]},\"type\":\"ConnectorPlacement.EquallySpacedConnector\",\"uuid\":\"c9b0d122-031a-4b9b-b90c-c03d042c7b1a\"}],\"packageUris\":[\"http://schema.mathworks.com/mf0/Connector/R2020b\"],\"version\":\"1.0\"}"
  udc(+) : PMIOPort  Side=Left
  uac(+) : PMIOPort  Port=2  Side=Right
  uac(-) : PMIOPort  Port=3  Side=Right
  udc(-) : PMIOPort  Port=4  Side=Left
  Meassurement : Outport
  wires:
  [Gate_4] -> Switch_4/1(G)
  [Gate_3] -> Switch_3/1(G)
  [Gate_2] -> Switch_2/1(G)
  [Gate_1] -> Switch_1/1(G)
  [Ideal_Switch_Current_4] -> Bus Creator/8  "Ideal_Switch_Current_4"
  [Ideal_Switch_Voltage_4] -> Bus Creator/7  "Ideal_Switch_Voltage_4"
  [Ideal_Switch_Current_3] -> Bus Creator/6  "Ideal_Switch_Current_3"
  [Ideal_Switch_Voltage_3] -> Bus Creator/5  "Ideal_Switch_Voltage_3"
  [Ideal_Switch_Current_2] -> Bus Creator/4  "Ideal_Switch_Current_2"
  [Ideal_Switch_Voltage_2] -> Bus Creator/3  "Ideal_Switch_Voltage_2"
  [Ideal_Switch_Current_1] -> Bus Creator/2  "Ideal_Switch_Current_1"
  [Ideal_Switch_Voltage_1] -> Bus Creator/1  "Ideal_Switch_Voltage_1"
  Gate_signals/1 -> Bus Selector/1
  Bus Creator/1 -> Meassurement/1
  Bus Selector/1 -> [Gate_1]  "<gate_signal_1>"
  Bus Selector/2 -> [Gate_2]  "<gate_signal_2>"
  Bus Selector/3 -> [Gate_3]  "<gate_signal_3>"
  Bus Selector/4 -> [Gate_4]  "<gate_signal_4>"
  connections:
  Switch_2/RConn1 -- uac(-)/RConn1 -- Switch_4/LConn1
  Switch_1/LConn1 -- udc(+)/RConn1 -- Switch_2/LConn1
  Switch_4/RConn1 -- Switch_3/RConn1 -- udc(-)/RConn1
  Switch_1/RConn1 -- Switch_3/LConn1 -- uac(+)/RConn1

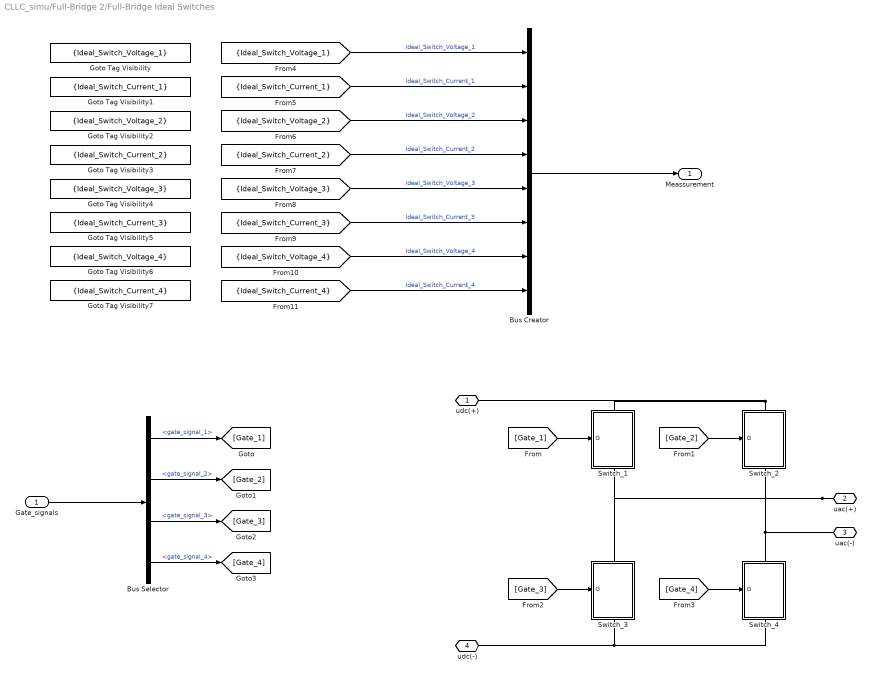
== system CLLC_simu/Full-Bridge 2/Full-Bridge Ideal Switches ==
  Gate_signals : Inport
  Bus Creator : BusCreator  Inputs=8
  Bus Selector : BusSelector  OutputSignals=gate_signal_1,gate_signal_2,gate_signal_3,gate_signal_4
  Goto Tag Visibility : GotoTagVisibility  GotoTag=Ideal_Switch_Voltage_1
  Goto Tag Visibility1 : GotoTagVisibility  GotoTag=Ideal_Switch_Current_1
  Goto Tag Visibility2 : GotoTagVisibility  GotoTag=Ideal_Switch_Voltage_2
  Goto Tag Visibility3 : GotoTagVisibility  GotoTag=Ideal_Switch_Current_2
  Goto Tag Visibility4 : GotoTagVisibility  GotoTag=Ideal_Switch_Voltage_3
  Goto Tag Visibility5 : GotoTagVisibility  GotoTag=Ideal_Switch_Current_3
  Goto Tag Visibility6 : GotoTagVisibility  GotoTag=Ideal_Switch_Voltage_4
  Goto Tag Visibility7 : GotoTagVisibility  GotoTag=Ideal_Switch_Current_4
  Switch_1 : Subsystem
      settings: PortSchema="{\"entries\":[{\"content\":{\"sides\":[{\"content\":{\"connectorIds\":[\"In1\"]},\"type\":\"ConnectorPlacement.EquallySpacedRectSide\",\"uuid\":\"812df248-72cf-4017-9d54-aef7207fce7f\"},{\"content\":{\"side\":\"RIGHT\"},\"type\":\"ConnectorPlacement.EquallySpacedRectSide\",\"uuid\":\"a66e31eb-6559-4312-afa0-26cb116d02bf\"},{\"content\":{\"connectorIds\":[\"LConn1\"],\"side\":\"TOP\"},\"type\":\"ConnectorPlacement.EquallySpacedRectSide\",\"uuid\":\"1df6feb4-8a8d-441a-a0dc-721a2bb21abb\"},{\"content\":{\"connectorIds\":[\"RConn1\"],\"side\":\"BOTTOM\"},\"type\":\"ConnectorPlacement.EquallySpacedRectSide\",\"uuid\":\"258c1e92-2fe7-4acf-9dd0-9c6d3fd42034\"}]},\"type\":\"ConnectorPlacement.EquallySpacedConnector\",\"uuid\":\"c9b0d122-031a-4b9b-b90c-c03d042c7b1a\"}],\"packageUris\":[\"http://schema.mathworks.com/mf0/Connector/R2020b\"],\"version\":\"1.0\"}"
  Switch_2 : Subsystem
      settings: PortSchema="{\"entries\":[{\"content\":{\"sides\":[{\"content\":{\"connectorIds\":[\"In1\"]},\"type\":\"ConnectorPlacement.EquallySpacedRectSide\",\"uuid\":\"812df248-72cf-4017-9d54-aef7207fce7f\"},{\"content\":{\"side\":\"RIGHT\"},\"type\":\"ConnectorPlacement.EquallySpacedRectSide\",\"uuid\":\"a66e31eb-6559-4312-afa0-26cb116d02bf\"},{\"content\":{\"connectorIds\":[\"LConn1\"],\"side\":\"TOP\"},\"type\":\"ConnectorPlacement.EquallySpacedRectSide\",\"uuid\":\"1df6feb4-8a8d-441a-a0dc-721a2bb21abb\"},{\"content\":{\"connectorIds\":[\"RConn1\"],\"side\":\"BOTTOM\"},\"type\":\"ConnectorPlacement.EquallySpacedRectSide\",\"uuid\":\"258c1e92-2fe7-4acf-9dd0-9c6d3fd42034\"}]},\"type\":\"ConnectorPlacement.EquallySpacedConnector\",\"uuid\":\"c9b0d122-031a-4b9b-b90c-c03d042c7b1a\"}],\"packageUris\":[\"http://schema.mathworks.com/mf0/Connector/R2020b\"],\"version\":\"1.0\"}"
  Switch_3 : Subsystem
      settings: PortSchema="{\"entries\":[{\"content\":{\"sides\":[{\"content\":{\"connectorIds\":[\"In1\"]},\"type\":\"ConnectorPlacement.EquallySpacedRectSide\",\"uuid\":\"812df248-72cf-4017-9d54-aef7207fce7f\"},{\"content\":{\"side\":\"RIGHT\"},\"type\":\"ConnectorPlacement.EquallySpacedRectSide\",\"uuid\":\"a66e31eb-6559-4312-afa0-26cb116d02bf\"},{\"content\":{\"connectorIds\":[\"LConn1\"],\"side\":\"TOP\"},\"type\":\"ConnectorPlacement.EquallySpacedRectSide\",\"uuid\":\"1df6feb4-8a8d-441a-a0dc-721a2bb21abb\"},{\"content\":{\"connectorIds\":[\"RConn1\"],\"side\":\"BOTTOM\"},\"type\":\"ConnectorPlacement.EquallySpacedRectSide\",\"uuid\":\"258c1e92-2fe7-4acf-9dd0-9c6d3fd42034\"}]},\"type\":\"ConnectorPlacement.EquallySpacedConnector\",\"uuid\":\"c9b0d122-031a-4b9b-b90c-c03d042c7b1a\"}],\"packageUris\":[\"http://schema.mathworks.com/mf0/Connector/R2020b\"],\"version\":\"1.0\"}"
  Switch_4 : Subsystem
      settings: PortSchema="{\"entries\":[{\"content\":{\"sides\":[{\"content\":{\"connectorIds\":[\"In1\"]},\"type\":\"ConnectorPlacement.EquallySpacedRectSide\",\"uuid\":\"812df248-72cf-4017-9d54-aef7207fce7f\"},{\"content\":{\"side\":\"RIGHT\"},\"type\":\"ConnectorPlacement.EquallySpacedRectSide\",\"uuid\":\"a66e31eb-6559-4312-afa0-26cb116d02bf\"},{\"content\":{\"connectorIds\":[\"LConn1\"],\"side\":\"TOP\"},\"type\":\"ConnectorPlacement.EquallySpacedRectSide\",\"uuid\":\"1df6feb4-8a8d-441a-a0dc-721a2bb21abb\"},{\"content\":{\"connectorIds\":[\"RConn1\"],\"side\":\"BOTTOM\"},\"type\":\"ConnectorPlacement.EquallySpacedRectSide\",\"uuid\":\"258c1e92-2fe7-4acf-9dd0-9c6d3fd42034\"}]},\"type\":\"ConnectorPlacement.EquallySpacedConnector\",\"uuid\":\"c9b0d122-031a-4b9b-b90c-c03d042c7b1a\"}],\"packageUris\":[\"http://schema.mathworks.com/mf0/Connector/R2020b\"],\"version\":\"1.0\"}"
  udc(+) : PMIOPort  Side=Left
  uac(+) : PMIOPort  Port=2  Side=Right
  uac(-) : PMIOPort  Port=3  Side=Right
  udc(-) : PMIOPort  Port=4  Side=Left
  Meassurement : Outport
  wires:
  [Gate_4] -> Switch_4/1(G)
  [Gate_3] -> Switch_3/1(G)
  [Gate_2] -> Switch_2/1(G)
  [Gate_1] -> Switch_1/1(G)
  [Ideal_Switch_Current_4] -> Bus Creator/8  "Ideal_Switch_Current_4"
  [Ideal_Switch_Voltage_4] -> Bus Creator/7  "Ideal_Switch_Voltage_4"
  [Ideal_Switch_Current_3] -> Bus Creator/6  "Ideal_Switch_Current_3"
  [Ideal_Switch_Voltage_3] -> Bus Creator/5  "Ideal_Switch_Voltage_3"
  [Ideal_Switch_Current_2] -> Bus Creator/4  "Ideal_Switch_Current_2"
  [Ideal_Switch_Voltage_2] -> Bus Creator/3  "Ideal_Switch_Voltage_2"
  [Ideal_Switch_Current_1] -> Bus Creator/2  "Ideal_Switch_Current_1"
  [Ideal_Switch_Voltage_1] -> Bus Creator/1  "Ideal_Switch_Voltage_1"
  Gate_signals/1 -> Bus Selector/1
  Bus Creator/1 -> Meassurement/1
  Bus Selector/1 -> [Gate_1]  "<gate_signal_1>"
  Bus Selector/2 -> [Gate_2]  "<gate_signal_2>"
  Bus Selector/3 -> [Gate_3]  "<gate_signal_3>"
  Bus Selector/4 -> [Gate_4]  "<gate_signal_4>"
  connections:
  Switch_2/RConn1 -- Switch_4/LConn1 -- uac(-)/RConn1
  Switch_2/LConn1 -- Switch_1/LConn1 -- udc(+)/RConn1
  Switch_4/RConn1 -- udc(-)/RConn1 -- Switch_3/RConn1
  uac(+)/RConn1 -- Switch_1/RConn1 -- Switch_3/LConn1

== system CLLC_simu/Controller/Controller/Subsystem ==
  In1 : Inport
  Add : Sum  Inputs=+++
  Add1 : Sum  Inputs=-+
  Gain : Gain  Gain=0.5
  Gain1 : Gain  Gain=0.0009
  Saturation : Saturate
  Unit Delay : UnitDelay  SampleTime=-1  HasFrameUpgradeWarning=on
  Out1 : Outport
  wires:
  In1/1 -> Gain1/1, Gain/1
  Gain/1 -> Add1/1, Add/1
  Gain1/1 -> Add/2
  Unit Delay/1 -> Add/3
  Add1/1 -> Unit Delay/1
  Add/1 -> Saturation/1
  Saturation/1 -> Out1/1, Add1/2

== system CLLC_simu/Controller/PWM Generator/Deadtime ==
  note: bravo!
  y : Inport
  AND : Logic  IconShape=distinctive  AllPortsSameDT=off  OutDataTypeStr=boolean
  Constant10 : Constant  Value=0.5
  Data Type Conversion : DataTypeConversion  OutDataTypeStr=double  SaturateOnIntegerOverflow=off  RndMeth=Floor
  Data Type Conversion3 : DataTypeConversion  OutDataTypeStr=double  SaturateOnIntegerOverflow=off  RndMeth=Floor
  GreaterThan : RelationalOperator  Operator=>  OutDataTypeStr=boolean  RndMeth=Simplest  InputSameDT=off
  Transport Delay : TransportDelay  DelayTime=Td
  1 : Outport
  wires:
  GreaterThan/1 -> AND/1, Data Type Conversion3/1
  Constant10/1 -> GreaterThan/2
  y/1 -> GreaterThan/1
  Transport Delay/1 -> AND/2
  AND/1 -> Data Type Conversion/1
  Data Type Conversion3/1 -> Transport Delay/1
  Data Type Conversion/1 -> 1/1

== system CLLC_simu/Controller/PWM Generator/Deadtime1 ==
  note: bravo!
  y : Inport
  AND : Logic  IconShape=distinctive  AllPortsSameDT=off  OutDataTypeStr=boolean
  Constant10 : Constant  Value=0.5
  Data Type Conversion : DataTypeConversion  OutDataTypeStr=double  SaturateOnIntegerOverflow=off  RndMeth=Floor
  Data Type Conversion3 : DataTypeConversion  OutDataTypeStr=double  SaturateOnIntegerOverflow=off  RndMeth=Floor
  GreaterThan : RelationalOperator  Operator=>  OutDataTypeStr=boolean  RndMeth=Simplest  InputSameDT=off
  Transport Delay : TransportDelay  DelayTime=Td
  1 : Outport
  wires:
  Data Type Conversion/1 -> 1/1
  Data Type Conversion3/1 -> Transport Delay/1
  AND/1 -> Data Type Conversion/1
  Transport Delay/1 -> AND/2
  y/1 -> GreaterThan/1
  Constant10/1 -> GreaterThan/2
  GreaterThan/1 -> Data Type Conversion3/1, AND/1

== system CLLC_simu/Controller/PWM Generator/Deadtime2 ==
  note: bravo!
  y : Inport
  AND : Logic  IconShape=distinctive  AllPortsSameDT=off  OutDataTypeStr=boolean
  Constant10 : Constant  Value=0.5
  Data Type Conversion : DataTypeConversion  OutDataTypeStr=double  SaturateOnIntegerOverflow=off  RndMeth=Floor
  Data Type Conversion3 : DataTypeConversion  OutDataTypeStr=double  SaturateOnIntegerOverflow=off  RndMeth=Floor
  GreaterThan : RelationalOperator  Operator=>  OutDataTypeStr=boolean  RndMeth=Simplest  InputSameDT=off
  Transport Delay : TransportDelay  DelayTime=Td
  1 : Outport
  wires:
  GreaterThan/1 -> AND/1, Data Type Conversion3/1
  Constant10/1 -> GreaterThan/2
  y/1 -> GreaterThan/1
  Transport Delay/1 -> AND/2
  AND/1 -> Data Type Conversion/1
  Data Type Conversion3/1 -> Transport Delay/1
  Data Type Conversion/1 -> 1/1

== system CLLC_simu/Controller/PWM Generator/Deadtime3 ==
  note: bravo!
  y : Inport
  AND : Logic  IconShape=distinctive  AllPortsSameDT=off  OutDataTypeStr=boolean
  Constant10 : Constant  Value=0.5
  Data Type Conversion : DataTypeConversion  OutDataTypeStr=double  SaturateOnIntegerOverflow=off  RndMeth=Floor
  Data Type Conversion3 : DataTypeConversion  OutDataTypeStr=double  SaturateOnIntegerOverflow=off  RndMeth=Floor
  GreaterThan : RelationalOperator  Operator=>  OutDataTypeStr=boolean  RndMeth=Simplest  InputSameDT=off
  Transport Delay : TransportDelay  DelayTime=Td
  1 : Outport
  wires:
  GreaterThan/1 -> AND/1, Data Type Conversion3/1
  Constant10/1 -> GreaterThan/2
  y/1 -> GreaterThan/1
  Transport Delay/1 -> AND/2
  AND/1 -> Data Type Conversion/1
  Data Type Conversion3/1 -> Transport Delay/1
  Data Type Conversion/1 -> 1/1

== system CLLC_simu/Controller/PWM Generator/Deadtime4 ==
  note: bravo!
  y : Inport
  AND : Logic  IconShape=distinctive  AllPortsSameDT=off  OutDataTypeStr=boolean
  Constant10 : Constant  Value=0.5
  Data Type Conversion : DataTypeConversion  OutDataTypeStr=double  SaturateOnIntegerOverflow=off  RndMeth=Floor
  Data Type Conversion3 : DataTypeConversion  OutDataTypeStr=double  SaturateOnIntegerOverflow=off  RndMeth=Floor
  GreaterThan : RelationalOperator  Operator=>  OutDataTypeStr=boolean  RndMeth=Simplest  InputSameDT=off
  Transport Delay : TransportDelay  DelayTime=Td
  1 : Outport
  wires:
  Data Type Conversion/1 -> 1/1
  Data Type Conversion3/1 -> Transport Delay/1
  AND/1 -> Data Type Conversion/1
  Transport Delay/1 -> AND/2
  y/1 -> GreaterThan/1
  Constant10/1 -> GreaterThan/2
  GreaterThan/1 -> Data Type Conversion3/1, AND/1

== system CLLC_simu/Controller/PWM Generator/Deadtime5 ==
  note: bravo!
  y : Inport
  AND : Logic  IconShape=distinctive  AllPortsSameDT=off  OutDataTypeStr=boolean
  Constant10 : Constant  Value=0.5
  Data Type Conversion : DataTypeConversion  OutDataTypeStr=double  SaturateOnIntegerOverflow=off  RndMeth=Floor
  Data Type Conversion3 : DataTypeConversion  OutDataTypeStr=double  SaturateOnIntegerOverflow=off  RndMeth=Floor
  GreaterThan : RelationalOperator  Operator=>  OutDataTypeStr=boolean  RndMeth=Simplest  InputSameDT=off
  Transport Delay : TransportDelay  DelayTime=Td
  1 : Outport
  wires:
  GreaterThan/1 -> AND/1, Data Type Conversion3/1
  Constant10/1 -> GreaterThan/2
  y/1 -> GreaterThan/1
  Transport Delay/1 -> AND/2
  AND/1 -> Data Type Conversion/1
  Data Type Conversion3/1 -> Transport Delay/1
  Data Type Conversion/1 -> 1/1

== system CLLC_simu/Controller/PWM Generator/Deadtime6 ==
  note: bravo!
  y : Inport
  AND : Logic  IconShape=distinctive  AllPortsSameDT=off  OutDataTypeStr=boolean
  Constant10 : Constant  Value=0.5
  Data Type Conversion : DataTypeConversion  OutDataTypeStr=double  SaturateOnIntegerOverflow=off  RndMeth=Floor
  Data Type Conversion3 : DataTypeConversion  OutDataTypeStr=double  SaturateOnIntegerOverflow=off  RndMeth=Floor
  GreaterThan : RelationalOperator  Operator=>  OutDataTypeStr=boolean  RndMeth=Simplest  InputSameDT=off
  Transport Delay : TransportDelay  DelayTime=Td
  1 : Outport
  wires:
  Data Type Conversion/1 -> 1/1
  Data Type Conversion3/1 -> Transport Delay/1
  AND/1 -> Data Type Conversion/1
  Transport Delay/1 -> AND/2
  y/1 -> GreaterThan/1
  Constant10/1 -> GreaterThan/2
  GreaterThan/1 -> Data Type Conversion3/1, AND/1

== system CLLC_simu/Controller/PWM Generator/Deadtime7 ==
  note: bravo!
  y : Inport
  AND : Logic  IconShape=distinctive  AllPortsSameDT=off  OutDataTypeStr=boolean
  Constant10 : Constant  Value=0.5
  Data Type Conversion : DataTypeConversion  OutDataTypeStr=double  SaturateOnIntegerOverflow=off  RndMeth=Floor
  Data Type Conversion3 : DataTypeConversion  OutDataTypeStr=double  SaturateOnIntegerOverflow=off  RndMeth=Floor
  GreaterThan : RelationalOperator  Operator=>  OutDataTypeStr=boolean  RndMeth=Simplest  InputSameDT=off
  Transport Delay : TransportDelay  DelayTime=Td
  1 : Outport
  wires:
  GreaterThan/1 -> AND/1, Data Type Conversion3/1
  Constant10/1 -> GreaterThan/2
  y/1 -> GreaterThan/1
  Transport Delay/1 -> AND/2
  AND/1 -> Data Type Conversion/1
  Data Type Conversion3/1 -> Transport Delay/1
  Data Type Conversion/1 -> 1/1

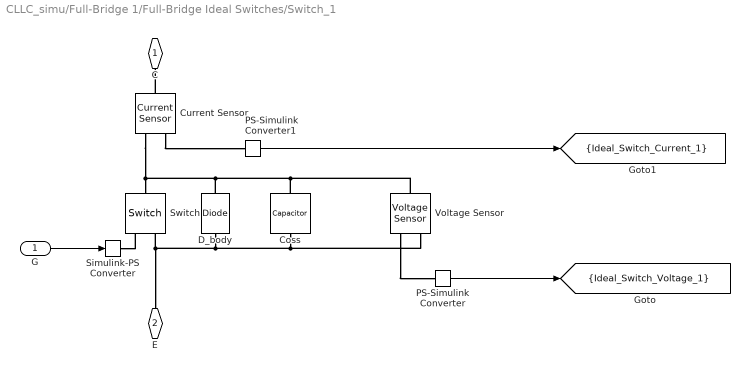
== system CLLC_simu/Full-Bridge 1/Full-Bridge Ideal Switches/Switch_1 ==
  G : Inport
  Coss : fl_lib/Electrical/Electrical Elements/Capacitor  c=1e-9 F  r=1e-6 Ohm  g=0 1/Ohm  i_specify=off  i_priority=None  i=0 A  i_nominal_specify=off  i_nominal_value=1  i_nominal_unit=A  v_specify=off  v_priority=None  v=0 V  v_nominal_specify=off  v_nominal_value=1  v_nominal_unit=V  vc_specify=off  vc_priority=High  vc=0 V  vc_nominal_specify=off  vc_nominal_value=1  vc_nominal_unit=V
  Current Sensor : fl_lib/Electrical/Electrical Sensors/Current Sensor
  D_body : fl_lib/Electrical/Electrical Elements/Diode  Vf=0.6 V  Ron=15e-4 Ohm  Goff=1e-8 1/Ohm  i_specify=off  i_priority=None  i=0 A  i_nominal_specify=off  i_nominal_value=1  i_nominal_unit=A  v_specify=off  v_priority=None  v=0 V  v_nominal_specify=off  v_nominal_value=1  v_nominal_unit=V
  PS-Simulink Converter : nesl_utility/PS-Simulink Converter  PhysicalDomain=network_engine_domain  SubClassName=ps_output  LeftPortType=input  RightPortType=output  PseudoPeriodic=off  Frequencies=[]  VectorFormat=inherit  Unit=inherit  AffineConversion=off
  PS-Simulink Converter1 : nesl_utility/PS-Simulink Converter  PhysicalDomain=network_engine_domain  SubClassName=ps_output  LeftPortType=input  RightPortType=output  PseudoPeriodic=off  Frequencies=[]  VectorFormat=inherit  Unit=inherit  AffineConversion=off
  Simulink-PS Converter : nesl_utility/Simulink-PS Converter  PhysicalDomain=network_engine_domain  SubClassName=ps_input  LeftPortType=input  RightPortType=output  PseudoPeriodic=off  Frequencies=[]  NoiseDistribution=none  NoiseParameters=[]  Unit=1  AffineConversion=off  FilteringAndDerivatives=provide  SimscapeFilterOrder=1  InputFilterTimeConstant=0.001  UdotUserProvided=0
  Switch : fl_lib/Electrical/Electrical Elements/Switch  R_closed=0.01 Ohm  G_open=1e-8 1/Ohm  Threshold=0.5  i_specify=off  i_priority=None  i=0 A  i_nominal_specify=off  i_nominal_value=1  i_nominal_unit=A  v_specify=off  v_priority=None  v=0 V  v_nominal_specify=off  v_nominal_value=1  v_nominal_unit=V
  Voltage Sensor : fl_lib/Electrical/Electrical Sensors/Voltage Sensor
  C : PMIOPort  Side=Left
  E : PMIOPort  Port=2  Side=Right
  tag scope: Ideal_Switch_Current_1=scoped, Ideal_Switch_Voltage_1=scoped
  wires:
  G/1 -> Simulink-PS Converter/1
  PS-Simulink Converter/1 -> [Ideal_Switch_Voltage_1]
  PS-Simulink Converter1/1 -> [Ideal_Switch_Current_1]
  connections:
  D_body/LConn1 -- Voltage Sensor/RConn2 -- Coss/RConn1 -- E/RConn1 -- Switch/RConn2
  D_body/RConn1 -- Voltage Sensor/LConn1 -- Coss/LConn1 -- Current Sensor/RConn2 -- Switch/LConn1
  Simulink-PS Converter/RConn1 -- Switch/RConn1
  Voltage Sensor/RConn1 -- PS-Simulink Converter/LConn1
  Current Sensor/LConn1 -- C/RConn1
  Current Sensor/RConn1 -- PS-Simulink Converter1/LConn1

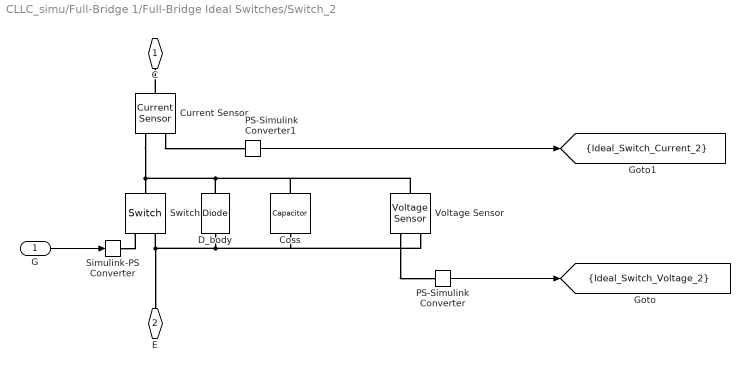
== system CLLC_simu/Full-Bridge 1/Full-Bridge Ideal Switches/Switch_2 ==
  G : Inport
  Coss : fl_lib/Electrical/Electrical Elements/Capacitor  c=1e-9 F  r=1e-6 Ohm  g=0 1/Ohm  i_specify=off  i_priority=None  i=0 A  i_nominal_specify=off  i_nominal_value=1  i_nominal_unit=A  v_specify=off  v_priority=None  v=0 V  v_nominal_specify=off  v_nominal_value=1  v_nominal_unit=V  vc_specify=off  vc_priority=High  vc=0 V  vc_nominal_specify=off  vc_nominal_value=1  vc_nominal_unit=V
  Current Sensor : fl_lib/Electrical/Electrical Sensors/Current Sensor
  D_body : fl_lib/Electrical/Electrical Elements/Diode  Vf=0.6 V  Ron=15e-4 Ohm  Goff=1e-8 1/Ohm  i_specify=off  i_priority=None  i=0 A  i_nominal_specify=off  i_nominal_value=1  i_nominal_unit=A  v_specify=off  v_priority=None  v=0 V  v_nominal_specify=off  v_nominal_value=1  v_nominal_unit=V
  PS-Simulink Converter : nesl_utility/PS-Simulink Converter  PhysicalDomain=network_engine_domain  SubClassName=ps_output  LeftPortType=input  RightPortType=output  PseudoPeriodic=off  Frequencies=[]  VectorFormat=inherit  Unit=inherit  AffineConversion=off
  PS-Simulink Converter1 : nesl_utility/PS-Simulink Converter  PhysicalDomain=network_engine_domain  SubClassName=ps_output  LeftPortType=input  RightPortType=output  PseudoPeriodic=off  Frequencies=[]  VectorFormat=inherit  Unit=inherit  AffineConversion=off
  Simulink-PS Converter : nesl_utility/Simulink-PS Converter  PhysicalDomain=network_engine_domain  SubClassName=ps_input  LeftPortType=input  RightPortType=output  PseudoPeriodic=off  Frequencies=[]  NoiseDistribution=none  NoiseParameters=[]  Unit=1  AffineConversion=off  FilteringAndDerivatives=provide  SimscapeFilterOrder=1  InputFilterTimeConstant=0.001  UdotUserProvided=0
  Switch : fl_lib/Electrical/Electrical Elements/Switch  R_closed=0.01 Ohm  G_open=1e-8 1/Ohm  Threshold=0.5  i_specify=off  i_priority=None  i=0 A  i_nominal_specify=off  i_nominal_value=1  i_nominal_unit=A  v_specify=off  v_priority=None  v=0 V  v_nominal_specify=off  v_nominal_value=1  v_nominal_unit=V
  Voltage Sensor : fl_lib/Electrical/Electrical Sensors/Voltage Sensor
  C : PMIOPort  Side=Left
  E : PMIOPort  Port=2  Side=Right
  tag scope: Ideal_Switch_Current_2=scoped, Ideal_Switch_Voltage_2=scoped
  wires:
  PS-Simulink Converter1/1 -> [Ideal_Switch_Current_2]
  PS-Simulink Converter/1 -> [Ideal_Switch_Voltage_2]
  G/1 -> Simulink-PS Converter/1
  connections:
  Current Sensor/RConn1 -- PS-Simulink Converter1/LConn1
  Current Sensor/LConn1 -- C/RConn1
  Voltage Sensor/RConn1 -- PS-Simulink Converter/LConn1
  Simulink-PS Converter/RConn1 -- Switch/RConn1
  Current Sensor/RConn2 -- Switch/LConn1 -- D_body/RConn1 -- Coss/LConn1 -- Voltage Sensor/LConn1
  Coss/RConn1 -- Voltage Sensor/RConn2 -- D_body/LConn1 -- Switch/RConn2 -- E/RConn1

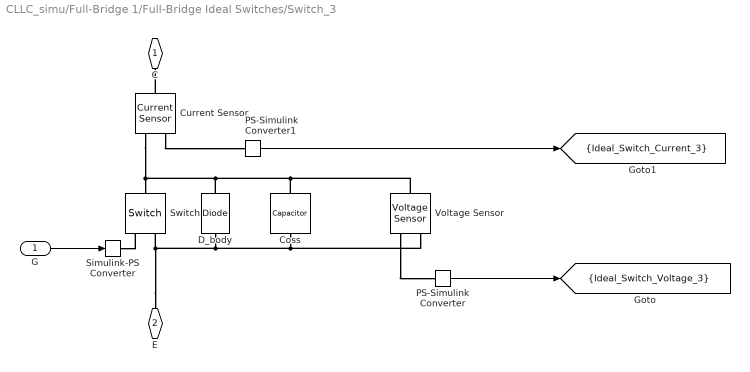
== system CLLC_simu/Full-Bridge 1/Full-Bridge Ideal Switches/Switch_3 ==
  G : Inport
  Coss : fl_lib/Electrical/Electrical Elements/Capacitor  c=1e-9 F  r=1e-6 Ohm  g=0 1/Ohm  i_specify=off  i_priority=None  i=0 A  i_nominal_specify=off  i_nominal_value=1  i_nominal_unit=A  v_specify=off  v_priority=None  v=0 V  v_nominal_specify=off  v_nominal_value=1  v_nominal_unit=V  vc_specify=off  vc_priority=High  vc=0 V  vc_nominal_specify=off  vc_nominal_value=1  vc_nominal_unit=V
  Current Sensor : fl_lib/Electrical/Electrical Sensors/Current Sensor
  D_body : fl_lib/Electrical/Electrical Elements/Diode  Vf=0.6 V  Ron=15e-4 Ohm  Goff=1e-8 1/Ohm  i_specify=off  i_priority=None  i=0 A  i_nominal_specify=off  i_nominal_value=1  i_nominal_unit=A  v_specify=off  v_priority=None  v=0 V  v_nominal_specify=off  v_nominal_value=1  v_nominal_unit=V
  PS-Simulink Converter : nesl_utility/PS-Simulink Converter  PhysicalDomain=network_engine_domain  SubClassName=ps_output  LeftPortType=input  RightPortType=output  PseudoPeriodic=off  Frequencies=[]  VectorFormat=inherit  Unit=inherit  AffineConversion=off
  PS-Simulink Converter1 : nesl_utility/PS-Simulink Converter  PhysicalDomain=network_engine_domain  SubClassName=ps_output  LeftPortType=input  RightPortType=output  PseudoPeriodic=off  Frequencies=[]  VectorFormat=inherit  Unit=inherit  AffineConversion=off
  Simulink-PS Converter : nesl_utility/Simulink-PS Converter  PhysicalDomain=network_engine_domain  SubClassName=ps_input  LeftPortType=input  RightPortType=output  PseudoPeriodic=off  Frequencies=[]  NoiseDistribution=none  NoiseParameters=[]  Unit=1  AffineConversion=off  FilteringAndDerivatives=provide  SimscapeFilterOrder=1  InputFilterTimeConstant=0.001  UdotUserProvided=0
  Switch : fl_lib/Electrical/Electrical Elements/Switch  R_closed=0.01 Ohm  G_open=1e-8 1/Ohm  Threshold=0.5  i_specify=off  i_priority=None  i=0 A  i_nominal_specify=off  i_nominal_value=1  i_nominal_unit=A  v_specify=off  v_priority=None  v=0 V  v_nominal_specify=off  v_nominal_value=1  v_nominal_unit=V
  Voltage Sensor : fl_lib/Electrical/Electrical Sensors/Voltage Sensor
  C : PMIOPort  Side=Left
  E : PMIOPort  Port=2  Side=Right
  tag scope: Ideal_Switch_Current_3=scoped, Ideal_Switch_Voltage_3=scoped
  wires:
  G/1 -> Simulink-PS Converter/1
  PS-Simulink Converter/1 -> [Ideal_Switch_Voltage_3]
  PS-Simulink Converter1/1 -> [Ideal_Switch_Current_3]
  connections:
  E/RConn1 -- Switch/RConn2 -- D_body/LConn1 -- Voltage Sensor/RConn2 -- Coss/RConn1
  Voltage Sensor/LConn1 -- Coss/LConn1 -- D_body/RConn1 -- Switch/LConn1 -- Current Sensor/RConn2
  Simulink-PS Converter/RConn1 -- Switch/RConn1
  Voltage Sensor/RConn1 -- PS-Simulink Converter/LConn1
  Current Sensor/LConn1 -- C/RConn1
  Current Sensor/RConn1 -- PS-Simulink Converter1/LConn1
